simulink model "LCL_lcl_inverter"  (R2017b)
settings: Solver=ode23  StartTime=0.0  StopTime=0.03  MaxStep=1e-4  RelTol=1e-3
InitFcn:
  | %%%%系统参数
  | f = 85000;
  | w = 2*pi*f;
  | Vdc = 200;
  | Up = 0.9*Vdc;
  | 
  | %%%%%线圈参数
  | Ltp = 263e-6;
  | Lts = 258e-6;
  | %%%线圈互感
  | M = 60e-6;
  | 
  | Iout = 16;
  | 
  | Lp1 = sqrt(Up*Mta)/sqrt(Iout*w);
  | Ctp = 1/(4*pi^2*f^2*(Ltp-Lp1));
  | Cp1 = 1/(4*pi^2*f^2*Lp1);
  | 
  | Lp2 = sqrt(Up*Mta)/sqrt(Iout*w);
  | Cts = 1/(4*pi^2*f^2*(Lts-Lp2));
  | Cp2 = 1/(4*pi^2*f^2*Lp2);
undefined symbols (not defined in the file): Cz, Lp, Lz
libraries: powerlib x26, peRmsMeasurement x11, simulink x2, powerlib_meascontrol x2
settings Model: Creator=余杰  LastModifiedBy=SuperWindows
settings DebuggingCC: UnconnectedInputMsg=none  UnconnectedOutputMsg=none  UnconnectedLineMsg=none

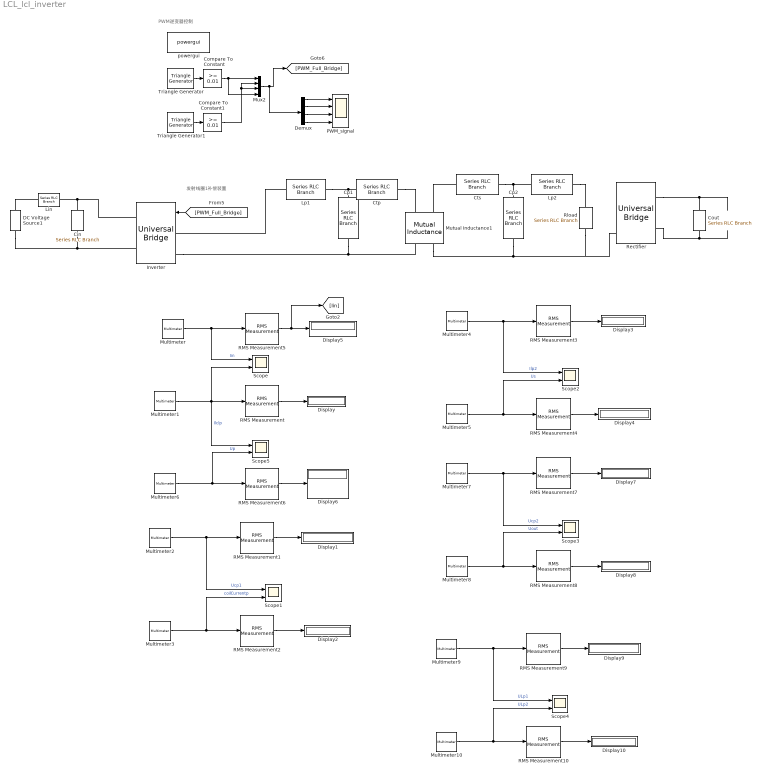
== system LCL_lcl_inverter ==
  note: PWM逆变器控制
  note: 发射线圈1补偿装置
  Cin : powerlib/Elements/Series RLC Branch  LConnTagsString=__new0  RConnTagsString=__new0  BranchType=RC  Resistance=0.1  Inductance=Lz  SetiL0=off  InitialCurrent=0  Capacitance=10e-6  Setx0=off  InitialVoltage=0  Measurements=Branch voltage and current
  Compare To Constant : simulink/Logic and Bit Operations/Compare To Constant  relop=>=  const=0.01  OutDataTypeStr=boolean
  Compare To Constant1 : simulink/Logic and Bit Operations/Compare To Constant  relop=>=  const=0.01  OutDataTypeStr=boolean
  Cout : powerlib/Elements/Series RLC Branch  LConnTagsString=__new0  RConnTagsString=__new0  BranchType=C  Resistance=5  Inductance=10e-3  SetiL0=off  InitialCurrent=0  Capacitance=470e-6*2  Setx0=off  InitialVoltage=0  Measurements=None
  Cp1 : powerlib/Elements/Series RLC Branch  LConnTagsString=__new0  RConnTagsString=__new0  BranchType=C  Resistance=1  Inductance=Lp  SetiL0=off  InitialCurrent=0  Capacitance=Cp1  Setx0=off  InitialVoltage=0  Measurements=Branch voltage and current
  Cp2 : powerlib/Elements/Series RLC Branch  LConnTagsString=__new0  RConnTagsString=__new0  BranchType=C  Resistance=1  Inductance=Lp  SetiL0=off  InitialCurrent=0  Capacitance=Cp2  Setx0=off  InitialVoltage=0  Measurements=Branch voltage and current
  Ctp : powerlib/Elements/Series RLC Branch  LConnTagsString=__new0  RConnTagsString=__new0  BranchType=C  Resistance=1  Inductance=Lp  SetiL0=off  InitialCurrent=0  Capacitance=Ctp  Setx0=off  InitialVoltage=0  Measurements=Branch voltage and current
  Cts : powerlib/Elements/Series RLC Branch  LConnTagsString=__new0  RConnTagsString=__new0  BranchType=C  Resistance=1  Inductance=Lp  SetiL0=off  InitialCurrent=0  Capacitance=Cts  Setx0=off  InitialVoltage=0  Measurements=Branch voltage and current
  DC Voltage Source1 : powerlib/Electrical Sources/DC Voltage Source  Amplitude=200  Measurements=None
  Demux : Demux
  Display{,1..10} (11 alike) : Display
  "Inverter " : powerlib/Power Electronics/Universal Bridge  Arms=2  SnubberResistance=1e6  SnubberCapacitance=inf  Device=MOSFET / Diodes  Ron=1e-3  Lon=0  ForwardVoltages="[  0  0  ]"  ForwardVoltage=0  GTOparameters=[ 10e-6 , 20e-6 ]  IGBTparameters=[ 1e-6 , 2e-6 ]  Measurements=All voltages and currents  Measurements_2=None  converterType=Rectifier
  Lin : powerlib/Elements/Series RLC Branch  LConnTagsString=__new0  RConnTagsString=__new0  BranchType=L  Resistance=1  Inductance=10e-6  SetiL0=off  InitialCurrent=0  Capacitance=Cz  Setx0=off  InitialVoltage=0  Measurements=Branch voltage and current
  Lp1 : powerlib/Elements/Series RLC Branch  LConnTagsString=__new0  RConnTagsString=__new0  BranchType=L  Resistance=1  Inductance=Lp1  SetiL0=off  InitialCurrent=0  Capacitance=1e-6  Setx0=off  InitialVoltage=0  Measurements=Branch voltage and current
  Lp2 : powerlib/Elements/Series RLC Branch  LConnTagsString=__new0  RConnTagsString=__new0  BranchType=L  Resistance=1  Inductance=Lp2  SetiL0=off  InitialCurrent=0  Capacitance=1e-6  Setx0=off  InitialVoltage=0  Measurements=Branch voltage and current
  Multimeter : powerlib/Measurements/Multimeter  PhasorSimulation=off  OutputType=Complex  sel=29  L=42  Gain=1  yselected={'Ib: Lin'};  PSBOutputType=1  PSBequivalent=0  AxesSetting=[0,0.1,-100,100]  Display=0  SavedBlockNames=-11
  Multimeter1 : powerlib/Measurements/Multimeter  PhasorSimulation=off  OutputType=Complex  sel=32  L=42  Gain=1  yselected={'Ib: Lp1'};  PSBOutputType=1  PSBequivalent=0  AxesSetting=[0,0.1,-100,100]  Display=0  SavedBlockNames=-11
  Multimeter10 : powerlib/Measurements/Multimeter  PhasorSimulation=off  OutputType=Complex  sel=8  L=42  Gain=1  yselected={'Ub: Lp2'};  PSBOutputType=1  PSBequivalent=0  AxesSetting=[0,0.1,-100,100]  Display=0  SavedBlockNames=-11
  Multimeter2 : powerlib/Measurements/Multimeter  PhasorSimulation=off  OutputType=Complex  sel=3  L=42  Gain=1  yselected={'Ub: Cp1'};  PSBOutputType=1  PSBequivalent=0  AxesSetting=[0,0.1,-100,100]  Display=0  SavedBlockNames=-11
  Multimeter3 : powerlib/Measurements/Multimeter  PhasorSimulation=off  OutputType=Complex  sel=33  L=42  Gain=1  yselected={'Iw1: Mutual Inductance1'};  PSBOutputType=1  PSBequivalent=0  AxesSetting=[0,0.1,-100,100]  Display=0  SavedBlockNames=-11
  Multimeter4 : powerlib/Measurements/Multimeter  PhasorSimulation=off  OutputType=Complex  sel=31  L=42  Gain=1  yselected={'Ib: Lp2'};  PSBOutputType=1  PSBequivalent=0  AxesSetting=[0,0.1,-100,100]  Display=0  SavedBlockNames=-11
  Multimeter5 : powerlib/Measurements/Multimeter  PhasorSimulation=off  OutputType=Complex  sel=16  L=42  Gain=1  yselected={'Uab: Rectifier'};  PSBOutputType=1  PSBequivalent=0  AxesSetting=[0,0.1,-100,100]  Display=0  SavedBlockNames=-11
  Multimeter6 : powerlib/Measurements/Multimeter  PhasorSimulation=off  OutputType=Complex  sel=22  L=42  Gain=1  yselected={'Uab: Inverter '};  PSBOutputType=1  PSBequivalent=0  AxesSetting=[0,0.1,-100,100]  Display=0  SavedBlockNames=-11
  Multimeter7 : powerlib/Measurements/Multimeter  PhasorSimulation=off  OutputType=Complex  sel=2  L=42  Gain=1  yselected={'Ub: Cp2'};  PSBOutputType=1  PSBequivalent=0  AxesSetting=[0,0.1,-100,100]  Display=0  SavedBlockNames=-11
  Multimeter8 : powerlib/Measurements/Multimeter  PhasorSimulation=off  OutputType=Complex  sel=7  L=42  Gain=1  yselected={'Ub: Rload'};  PSBOutputType=1  PSBequivalent=0  AxesSetting=[0,0.1,-100,100]  Display=0  SavedBlockNames=-11
  Multimeter9 : powerlib/Measurements/Multimeter  PhasorSimulation=off  OutputType=Complex  sel=9  L=42  Gain=1  yselected={'Ub: Lp1'};  PSBOutputType=1  PSBequivalent=0  AxesSetting=[0,0.1,-100,100]  Display=0  SavedBlockNames=-11
  Mutual Inductance1 : powerlib/Elements/Mutual Inductance  LConnTagsString=a|b  RConnTagsString=A|B  TypeOfMutual=Generalized mutual inductance  NumberOfWindings=2  SelfImpedance1=[0.001 1e-03]  SelfImpedance2=[0.001 1e-03]  ThreeWindings=off  SelfImpedance3=[ 1.1 1.1e-03]  MutualImpedance=[0 50e-06]  InductanceMatrix=[Ltp M;M Lts]  ResistanceMatrix="[0.001 0 ;  0 0.001]"  Measurements=Winding voltages and currents
      settings: AttributesFormatString=\n  SourceProductName=Simscape Power Systems  SourceProductBaseCode=PS
  Mux2 : Mux
  PWM_signal : Scope  NumInputPorts=4
  RMS Measurement{,1..4,7..10} (9 alike) : peRmsMeasurement/RMS Measurement  OverrideUsingVariant=Total  F=f  SpecifyHarmonics=off  K=[0 1 2]  Ts=0
  RMS Measurement5 : peRmsMeasurement/RMS Measurement  OverrideUsingVariant=Total  F=f/10  SpecifyHarmonics=off  K=[0 1 2]  Ts=0
  RMS Measurement6 : peRmsMeasurement/RMS Measurement  OverrideUsingVariant=Harmonic  F=f  SpecifyHarmonics=on  K=[0 1 2]  Ts=0
  Rectifier : powerlib/Power Electronics/Universal Bridge  Arms=2  SnubberResistance=1e6  SnubberCapacitance=inf  Device=MOSFET / Diodes  Ron=1e-3  Lon=0  ForwardVoltages="[  0  0  ]"  ForwardVoltage=0.4  GTOparameters=[ 10e-6 , 20e-6 ]  IGBTparameters=[ 1e-6 , 2e-6 ]  Measurements=All voltages and currents  Measurements_2=None  converterType=Rectifier
  Rload : powerlib/Elements/Series RLC Branch  LConnTagsString=__new0  RConnTagsString=__new0  BranchType=R  Resistance=5  Inductance=10e-3  SetiL0=off  InitialCurrent=0  Capacitance=470e-6  Setx0=off  InitialVoltage=0  Measurements=Branch voltage and current
  Scope{,1..5} (6 alike) : Scope  NumInputPorts=2
  Triangle Generator : powerlib_meascontrol/Pulse & Signal Generators/Triangle Generator  Freq=f  Phase=180  Ts=0
  Triangle Generator1 : powerlib_meascontrol/Pulse & Signal Generators/Triangle Generator  Freq=f  Phase=0  Ts=0
  powergui : powerlib/powergui  Priority=1  SimulationMode=Discrete  SampleTime=1e-8  frequency=60  Iterations=50  frequencyindice=0  Pbase=100e6  ErrMax=1e-4  UnitsV=kV  UnitsW=MW  buscounter=0  FunctionMessages=off  echomessages=off  EnableUseOfTLC=off  CurrentSourceSwitches=off  DisableSnubberDevices=off  DisableRonSwitches=off  DisableVfSwitches=off  DisplayEquations=off  SolverType=Tustin/Backward Euler (TBE)  Interpol=off  ExternalGateDelay=off  methode=off  Ts=100  x0status=blocks  SPID=on  SwTol=0  HookPort=off  RestoreLinks=warning  ResistiveCurrentMeasurement=off  Frange=[0:2:500]  Ylog=off  Xlog=on  ShowGrid=off  save=off  variable=ZData  structure=0  ZoomFFT=off  StartTime=0.0  cycles=1  DisplayStyle=1  fundamental=60  FreqAxis=off  MaxFrequency=1000  frequencyindicesteady=1  RmsSteady=1  display=off
  wires:
  Demux/3 -> PWM_signal/3
  Compare To Constant/1 -> Mux2/4, Mux2/1
  Triangle Generator/1 -> Compare To Constant/1
  Triangle Generator1/1 -> Compare To Constant1/1
  Demux/1 -> PWM_signal/1
  Demux/2 -> PWM_signal/2
  Demux/4 -> PWM_signal/4
  [PWM_Full_Bridge] -> "Inverter "/1
  Mux2/1 -> [PWM_Full_Bridge], Demux/1
  Compare To Constant1/1 -> Mux2/3, Mux2/2
  RMS Measurement/1 -> Display/1
  RMS Measurement6/1 -> Display6/1
  Multimeter/1 -> Scope/1, RMS Measurement5/1  "Iin"
  RMS Measurement5/1 -> [Iin], Display5/1
  Multimeter6/1 -> Scope5/2, RMS Measurement6/1  "Up"
  Multimeter1/1 -> Scope/2, Scope5/1, RMS Measurement/1  "Ilclp"
  Multimeter2/1 -> Scope1/1, RMS Measurement1/1  "Ucp1"
  RMS Measurement1/1 -> Display1/1
  Multimeter3/1 -> Scope1/2, RMS Measurement2/1  "coilCurrentp"
  RMS Measurement2/1 -> Display2/1
  Multimeter5/1 -> Scope2/2, RMS Measurement4/1  "Us"
  RMS Measurement3/1 -> Display3/1
  Multimeter4/1 -> Scope2/1, RMS Measurement3/1  "Ilp2"
  RMS Measurement4/1 -> Display4/1
  RMS Measurement7/1 -> Display7/1
  Multimeter7/1 -> Scope3/1, RMS Measurement7/1  "Ucp2"
  Multimeter8/1 -> Scope3/2, RMS Measurement8/1  "Uout"
  RMS Measurement8/1 -> Display8/1
  Multimeter10/1 -> Scope4/2, RMS Measurement10/1  "ULp2"
  RMS Measurement9/1 -> Display9/1
  Multimeter9/1 -> Scope4/1, RMS Measurement9/1  "ULp1"
  RMS Measurement10/1 -> Display10/1
  connections:
  "Inverter "/LConn2 -- Cp1/RConn1 -- Mutual Inductance1/RConn1
  Rectifier/RConn1 -- Cout/LConn1
  Lp2/RConn1 -- Rload/LConn1
  Cout/RConn1 -- Rectifier/RConn2
  Lp1/LConn1 -- "Inverter "/LConn1
  DC Voltage Source1/LConn1 -- Cin/RConn1 -- "Inverter "/RConn2
  "Inverter "/RConn1 -- Lin/RConn1 -- Cin/LConn1
  DC Voltage Source1/RConn1 -- Lin/LConn1
  Ctp/RConn1 -- Mutual Inductance1/LConn1
  Cts/LConn1 -- Mutual Inductance1/LConn2
  Cts/RConn1 -- Cp2/LConn1 -- Lp2/LConn1
  Lp1/RConn1 -- Cp1/LConn1 -- Ctp/LConn1
  Cp2/RConn1 -- Rload/RConn1 -- Rectifier/LConn2 -- Mutual Inductance1/RConn2
